simulink model "hybrid_system_prog"  (Simulink 8.0)
settings: Solver=FixedStepDiscrete  StartTime=0.0  StopTime=10  FixedStep=sim_sample_time  RelTol=1e-6
undefined symbols (not defined in the file or in its folder): SysHybride
settings Model: Creator=bayoudh  LastModifiedBy=szabi  ExtModeAutoUpdateStatusClock=off
settings DataIOCC: SignalLoggingSaveFormat=ModelDataLogs
settings OptimizationCC: InitFltsAndDblsToZero=on
settings DebuggingCC: SaveWithParameterizedLinksMsg=none  FcnCallInpInsideContextMsg=UseLocalSettings  StrictBusMsg=Warning
settings SFSimCC: SimParseCustomCode=off
settings GRTTargetCC: TargetFcnLib=ansi_tfl_tmw.mat  CombineOutputUpdateFcns=off  GRTInterface=on

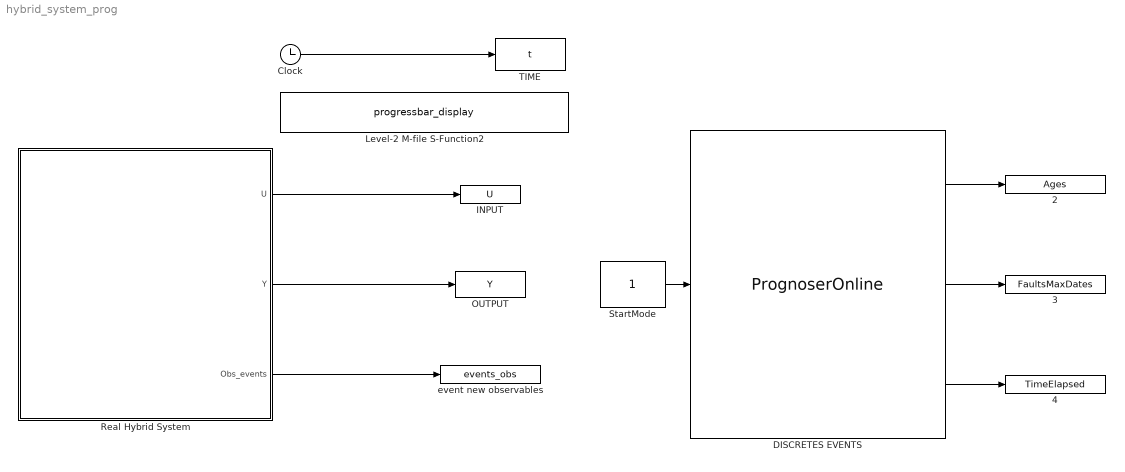
== system hybrid_system_prog ==
  2 : ToWorkspace  VariableName=Ages  SampleTime=-1
  3 : ToWorkspace  VariableName=FaultsMaxDates  SampleTime=-1
  4 : ToWorkspace  VariableName=TimeElapsed  SampleTime=-1
  Clock : Clock
  DISCRETES EVENTS : M-S-Function  FunctionName=PrognoserOnline
  INPUT : ToWorkspace  VariableName=U  SampleTime=-1
  Level-2 M-file S-Function2 : M-S-Function  FunctionName=progressbar_display
  OUTPUT : ToWorkspace  VariableName=Y  SampleTime=-1
  Real Hybrid System : Subsystem
  StartMode : Constant
  TIME : ToWorkspace  VariableName=t  SampleTime=-1
  event new observables : ToWorkspace  VariableName=events_obs  SampleTime=-1
  wires:
  Clock/1 -> TIME/1
  Real Hybrid System/1(U) -> INPUT/1
  Real Hybrid System/2(Y) -> OUTPUT/1
  Real Hybrid System/3(Obs_events) -> event new observables/1
  DISCRETES EVENTS/2 -> 3/1
  DISCRETES EVENTS/3 -> 4/1
  DISCRETES EVENTS/1 -> 2/1
  StartMode/1 -> DISCRETES EVENTS/1

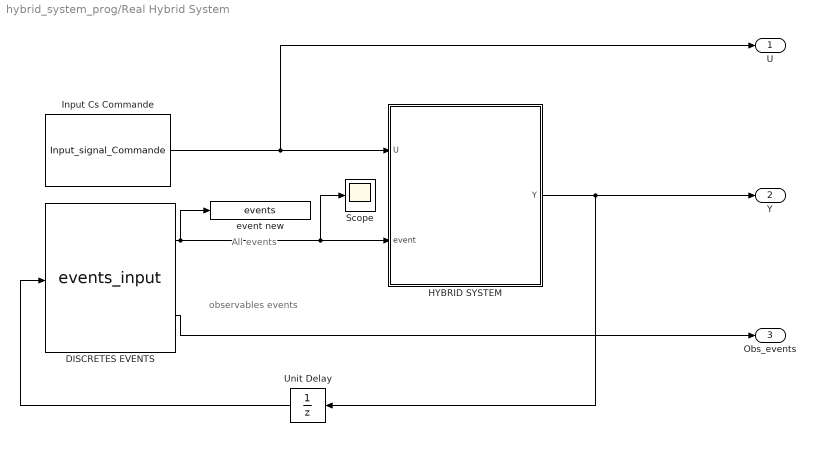
== system hybrid_system_prog/Real Hybrid System ==
  note: observables events
  note: All events
  DISCRETES EVENTS : M-S-Function  FunctionName=events_input
  HYBRID SYSTEM : Subsystem
  Input Cs Commande : S-Function  FunctionName=Input_signal_Commande  Parameters=rand(SysHybride('get_input_size'),1)*2*pi  EnableBusSupport=off
  Scope : Scope
  Unit Delay : UnitDelay  SampleTime=-1
  event new : ToWorkspace  VariableName=events  SampleTime=-1
  U : Outport
  Y : Outport  Port=2
  Obs_events : Outport  Port=3
  wires:
  Input Cs Commande/1 -> HYBRID SYSTEM/1(U), U/1
  HYBRID SYSTEM/1(Y) -> Y/1, Unit Delay/1
  DISCRETES EVENTS/1 -> event new/1, HYBRID SYSTEM/2(event), Scope/1
  DISCRETES EVENTS/2 -> Obs_events/1
  Unit Delay/1 -> DISCRETES EVENTS/1

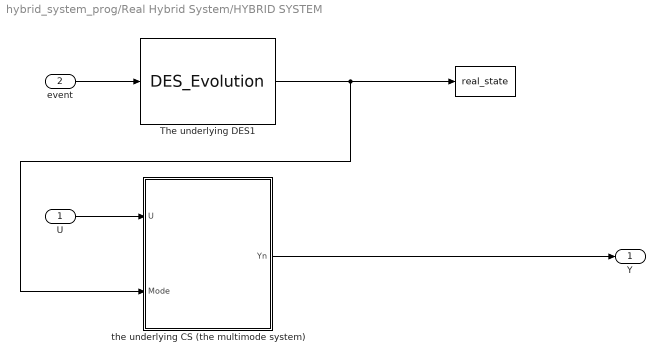
== system hybrid_system_prog/Real Hybrid System/HYBRID SYSTEM ==
  U : Inport
  event : Inport  Port=2
  "  " : ToWorkspace  VariableName=real_state  SampleTime=-1
  The underlying DES1 : S-Function  FunctionName=DES_Evolution  EnableBusSupport=off
  the underlying CS (the multimode system) : Subsystem
  Y : Outport
  wires:
  event/1 -> The underlying DES1/1
  U/1 -> the underlying CS (the multimode system)/1(U)
  The underlying DES1/1 -> the underlying CS (the multimode system)/2(Mode), "  "/1
  the underlying CS (the multimode system)/1(Yn) -> Y/1

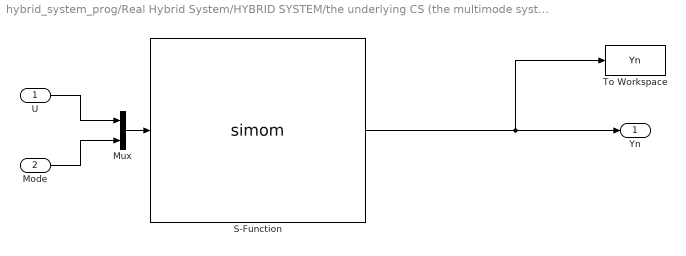
== system hybrid_system_prog/Real Hybrid System/HYBRID SYSTEM/the underlying CS (the multimode system) ==
  U : Inport
  Mode : Inport  Port=2
  Mux : Mux  Inputs=2
  S-Function : S-Function  FunctionName=simom  EnableBusSupport=off
  To Workspace : ToWorkspace  VariableName=Yn  SampleTime=-1
  Yn : Outport
  wires:
  S-Function/1 -> To Workspace/1, Yn/1
  U/1 -> Mux/1
  Mode/1 -> Mux/2
  Mux/1 -> S-Function/1
